simulink model "Final_Project"  (R2016b)
settings: Solver=ode1  StartTime=0.0  StopTime=30  FixedStep=ts  RelTol=1e-3  EnableMultiTasking=on
InitFcn:
  | ts = 0.01;
StartFcn:
  | %The GUI handles are by default hidden, turn them on
  | %set(0,'ShowHiddenHandles','on');
  | %Set up the arguments that will go into the gain block event callback listener
  | %blk = 'Final_Project/Angle';
  | %event = 'PostOutputs';
  | %listener = @updategui;
  | %Create the listener
  | %h = add_exec_event_listener(blk, event, listener);
  | ts = 0.01;
undefined symbols (not defined in the file or in its folder): Standard_Devices, UDP_Protocol
libraries: sldrtlib x2, ScienceStimHasomed_Lib x1, rtsync_lib x1
settings Model: Creator=Jan  LastModifiedBy=Jan
settings SolverCC: EnableConcurrentExecution=on
settings DataIOCC: SaveFormat=Array  SaveState=on  SignalLogging=off
settings OptimizationCC: BlockReduction=off  OptimizeBlockIOStorage=off  BufferReuse=off  GlobalBufferReuse=off  ExpressionFolding=off  LocalBlockOutputs=off
settings RTWCC: SystemTargetFile=sldrt.tlc  TemplateMakefile=sldrt.tmf  Description=Simulink Desktop Real-Time  RTWCompilerOptimization=on
settings CodeAppCC: MaxIdLength=95
settings SimulinkDesktopRealTimeCC: TargetPreCompLibLocation=C:\Program Files\MATLAB\R2016b\toolbox\sldrt\lib\win64  TargetLangStandard=C89/C90 (ANSI)  SupportVariableSizeSignals=off

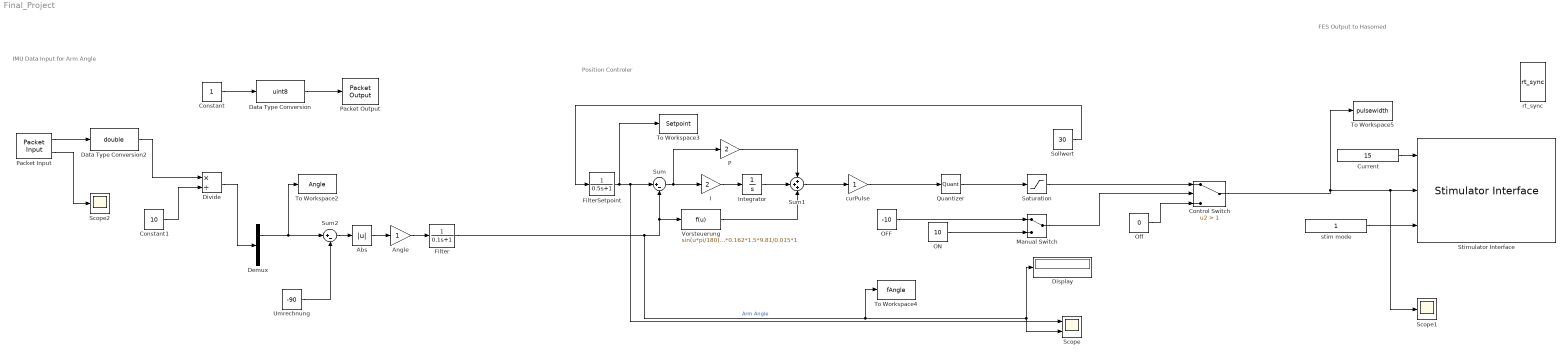
== system Final_Project ==
  note: FES Output to Hasomed
  note: Position Controler
  note: IMU Data Input for Arm Angle
  Abs : Abs
  Angle : Gain
  Constant : Constant
  Constant1 : Constant  Value=10
  Control Switch : Switch  Criteria=u2 > Threshold  Threshold=1
  Current : Constant  Value=15
  Data Type Conversion : DataTypeConversion  OutDataTypeStr=uint8
  Data Type Conversion2 : DataTypeConversion  OutDataTypeStr=double
  Demux : Demux  Outputs=6
  Display : Display
  Divide : Product  Inputs=*/
  Filter : TransferFcn  Denominator=[0.1 1]
  FilterSetpoint : TransferFcn  Denominator=[0.5 1]
  I : Gain  Gain=2
  Integrator : Integrator
  Manual Switch : ManualSwitch
  OFF : Constant  Value=-10
  ON : Constant  Value=10
  Off : Constant  Value=0
  P : Gain  Gain=2
  Packet Input : sldrtlib/Packet Input  SampleTime=ts  MaxMissedTicks=1000  ShowMissedTicks=on  YieldWhenWaiting=off  DrvName=Standard_Devices/UDP_Protocol  DrvAddress=4012  DrvOptions=[2130706433 8888]  PacketSize=12  DataTypes={'6*int16'}  ShowReady=off  ShowError=off  PacketID=1  ByteOrder=2  ShowTimestamp=off
      settings: AttributesFormatString=Standard Devices\nUDP Protocol [FACh]
  Packet Output : sldrtlib/Packet Output  SampleTime=ts  MaxMissedTicks=1000  ShowMissedTicks=on  YieldWhenWaiting=off  DrvName=Standard_Devices/UDP_Protocol  DrvAddress=4016  DrvOptions=[3232235954 8888]  PacketSize=1  DataTypes='int8'  ShowReady=off  ShowError=off  PacketID=1  ByteOrder=1  InitialValue=[]  FinalValue=[]
      settings: AttributesFormatString=Standard Devices\nUDP Protocol [FB0h]
  Quantizer : Quantizer  QuantizationInterval=10
  Saturation : Saturate  UpperLimit=400  LowerLimit=0
  Scope : Scope  NumInputPorts=2
  Scope1 : Scope
  Scope2 : Scope
  Sollwert : Constant  Value=30
  Stimulator Interface : ScienceStimHasomed_Lib/Stimulator Interface  Ts=ts  com_port=COM3  channelstim=1  tsone=20  tstwo=4  channellf=[]  nfactor=[]  outflag=on  dtflag=on
  Sum : Sum  Inputs=|+-
  Sum1 : Sum  Inputs=+++
  Sum2 : Sum  Inputs=|+-
  To Workspace2 : ToWorkspace  VariableName=Angle  SampleTime=-1
      settings: Save2DSignal=2-D array (concatenate along first dimension)
  To Workspace3 : ToWorkspace  VariableName=Setpoint  SampleTime=-1
      settings: Save2DSignal=2-D array (concatenate along first dimension)
  To Workspace4 : ToWorkspace  VariableName=fAngle  SampleTime=-1
      settings: Save2DSignal=2-D array (concatenate along first dimension)
  To Workspace5 : ToWorkspace  VariableName=pulsewidth  SampleTime=-1
      settings: Save2DSignal=2-D array (concatenate along first dimension)
  Umrechnung : Constant  Value=-90
  Vorsteuerung : Fcn  Expr=sin(u*pi/180)*0.162*1.5*9.81/0.015*1
  curPulse : Gain
  rt_sync : rtsync_lib/rt_sync  Ts=0.1  strict=off  outflag=on
  stim mode : Constant
  wires:
  Data Type Conversion/1 -> Packet Output/1
  Constant/1 -> Data Type Conversion/1
  Packet Input/1 -> Data Type Conversion2/1
  Constant1/1 -> Divide/2
  Quantizer/1 -> Saturation/1
  Off/1 -> Control Switch/3
  Current/1 -> Stimulator Interface/1
  stim mode/1 -> Stimulator Interface/3
  Control Switch/1 -> To Workspace5/1, Scope1/1, Stimulator Interface/2
  Saturation/1 -> Control Switch/1
  Filter/1 -> To Workspace4/1, Scope/2, Display/1, Vorsteuerung/1, Sum/2  "Arm Angle"
  Demux/2 -> Sum2/1, To Workspace2/1
  Umrechnung/1 -> Sum2/2
  Angle/1 -> Filter/1
  Data Type Conversion2/1 -> Divide/1
  Sum2/1 -> Abs/1
  Abs/1 -> Angle/1
  I/1 -> Integrator/1
  Sum/1 -> I/1, P/1
  P/1 -> Sum1/1
  Integrator/1 -> Sum1/2
  Sum1/1 -> curPulse/1
  curPulse/1 -> Quantizer/1
  Sollwert/1 -> FilterSetpoint/1
  FilterSetpoint/1 -> To Workspace3/1, Scope/1, Sum/1
  Manual Switch/1 -> Control Switch/2
  OFF/1 -> Manual Switch/1
  ON/1 -> Manual Switch/2
  Vorsteuerung/1 -> Sum1/3
  Divide/1 -> Demux/1
  Packet Input/2 -> Scope2/1
